simulink model "FuelC"  (R2019a)
settings: Solver=FixedStepDiscrete  StartTime=0.0  StopTime=102  FixedStep=1  RelTol=1e-3
libraries: simulink x1
settings Model: DataDictionary=fuelc.sldd  Creator=Admin  LastModifiedBy=Admin

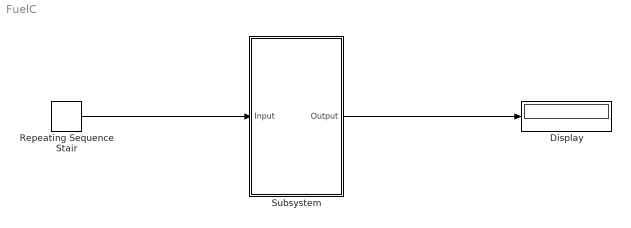
== system FuelC ==
  Display : Display
  Repeating Sequence Stair : simulink/Sources/Repeating Sequence Stair  OutValues=|  tsamp=-1  OutMin=[]  OutMax=[]  OutDataTypeStr=double  OutputDataTypeScalingMode=double  OutDataType=fixdt(0,8)  ConRadixGroup=Best Precision: Vector-wise  OutScaling=2^-12
      | [800
      | 1040
      | 1280
      | 1520
      | 1760
      | 2000
      | 2240
      | 2480
      | 2720
      | 2960
      | 3200
      | ].'
  Subsystem : Subsystem
  wires:
  Subsystem/1(Output) -> Display/1
  Repeating Sequence Stair/1 -> Subsystem/1(Input)

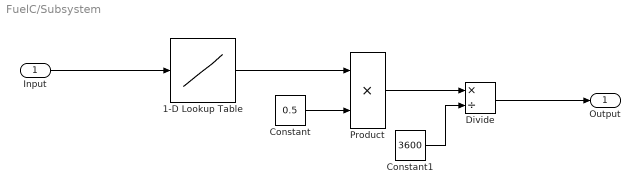
== system FuelC/Subsystem ==
  Input : Inport
  1-D Lookup Table : Lookup_n-D  NumberOfTableDimensions=1  LookupTableObject=''  BreakpointsForDimension1=|  BreakpointsForDimension1FirstPoint=10  BreakpointsForDimension2FirstPoint=10  BreakpointsForDimension1Spacing=12  BreakpointsForDimension2Spacing=12  IndexSearchMethod=Evenly spaced points  Table=|  InterpMethod=Flat  DiagnosticForOutOfRangeInput=Error  InternalRulePriority=Speed  RndMeth=Simplest  InputSameDT=on
      BreakpointsForDimension1=|
      | [800
      | 1040
      | 1280
      | 1520
      | 1760
      | 2000
      | 2240
      | 2480
      | 2720
      | 2960
      | 3200]
      Table=|
      | [18.33333333
      | 33.6375
      | 41.4
      | 49.1625
      | 56.925
      | 64.6875
      | 72.45
      | 80.2125
      | 87.975
      | 95.7375
      | 103.5
      | ]
  Constant : Constant  Value=0.5
  Constant1 : Constant  Value=3600
  Divide : Product  Inputs=*/
  Product : Product
  Output : Outport
  wires:
  1-D Lookup Table/1 -> Product/1
  Product/1 -> Divide/1
  Constant/1 -> Product/2
  Input/1 -> 1-D Lookup Table/1
  Divide/1 -> Output/1
  Constant1/1 -> Divide/2
